simulink model "Simulink_Beam_reduced"  (R2023a)
settings: Solver=VariableStepAuto  StartTime=0.0  StopTime=dur  RelTol=1e-6
values from neighbouring files (symbols this model uses):
  fsim = 0.5    [plots_NL.m]
libraries: cstblocks x1
settings Model: Creator=s128538  LastModifiedBy=mshakib
settings SolverCC: AlgebraicLoopSolver=TrustRegion
settings DataIOCC: ReturnWorkspaceOutputs=off
settings DebuggingCC: UnconnectedInputMsg=warning  UnconnectedOutputMsg=warning  UnconnectedLineMsg=warning  ArithmeticOperatorsInVariantConditions=warning
settings ModelReferenceCC: EnableRefExpFcnMdlSchedulingChecks=on
settings SFSimCC: SimUseLocalCustomCode=off  CustomCodeUndefinedFunction=UseInterfaceOnly
settings RTWCC: RTWUseLocalCustomCode=off

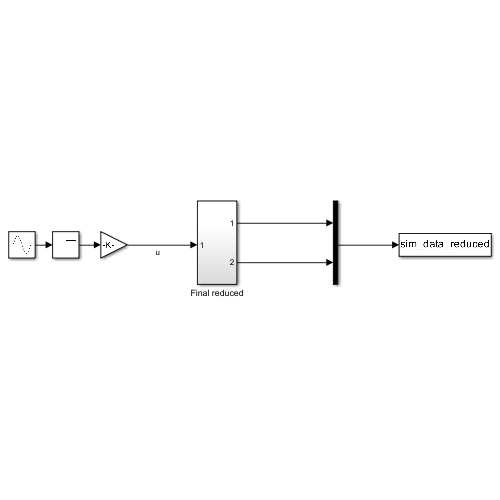
[thumbnail: Simulink's stored preview of the top-level diagram]
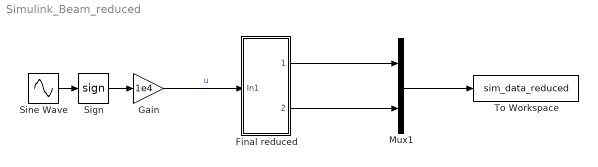
== system Simulink_Beam_reduced ==
  Final reduced : Subsystem
  Gain : Gain  Gain=1e4
  Mux1 : Mux  Inputs=2
  Sign : Signum
  Sine Wave : Sin  Frequency=2*pi*fsim  SampleTime=0
  To Workspace : ToWorkspace  VariableName=sim_data_reduced  SaveFormat=Timeseries  SampleTime=-1
  wires:
  Mux1/1 -> To Workspace/1
  Sign/1 -> Gain/1
  Final reduced/1(Out1) -> Mux1/1
  Final reduced/2(Out2) -> Mux1/2
  Sine Wave/1 -> Sign/1
  Gain/1 -> Final reduced/1(In1)  "u"

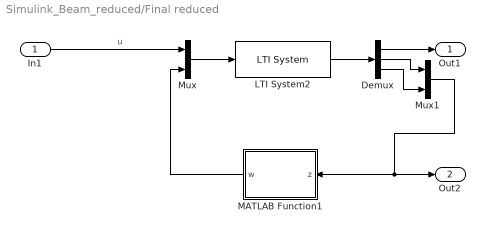
== system Simulink_Beam_reduced/Final reduced ==
  In1 : Inport
  Demux : Demux  Outputs=3
  LTI System2 : cstblocks/LTI System  sys=sys_red_final  IC=[]
  MATLAB Function1 : MATLAB Function  TreatAsAtomicUnit=on
  Mux : Mux  Inputs=2
  Mux1 : Mux  Inputs=2
  Out1 : Outport  VectorParamsAs1DForOutWhenUnconnected=off
  Out2 : Outport  Port=2  VectorParamsAs1DForOutWhenUnconnected=off
  wires:
  Mux/1 -> LTI System2/1
  LTI System2/1 -> Demux/1
  In1/1 -> Mux/1  "u"
  Demux/1 -> Out1/1
  Mux1/1 -> Out2/1, MATLAB Function1/1(z)
  Demux/3 -> Mux1/2
  Demux/2 -> Mux1/1
  MATLAB Function1/1(w) -> Mux/2

== matlab function Simulink_Beam_reduced/Final reduced/MATLAB Function1 ==
  data: z input; w output
function w = fcn(z)

w = [0;0];

w(1) = 2*(max(0,z(1))-z(1)/2);
w(2) = 2*(max(0,z(2))-z(2)/2);
